simulink model "MMC_SIMULATION (1)"  (R2024a)
settings: Solver=ode1  StartTime=0.0  StopTime=2  FixedStep=1e-5  MaxStep=1e-5  RelTol=1e-5  EnableMultiTasking=on
InitFcn:
  | tau_iac=ts_G_iac/4;                                         %Current loop speed
  | wAC=1/tau_iac;                                              %Frequency
  | L1AC=wAC/s;                                                 %Open loop IMC (L) transfer function to obtain a first order after closing the loop
  | Kp_AC=wAC*(Lg_1+La_1/2);                                    %Proportional constant of the controller
  | Ki_AC=wAC*(Rg_1+Ra_1/2);                                    %Integral constant of the controller
  | C_IMC_AC=(Kp_AC*s+Ki_AC)/s;                                 %IMC designed PI controller transfer function
  | TAC=minreal((C_IMC_AC)*G_iac/(1+(C_IMC_AC)*G_iac));         %Closed loop transfer function
  | 
  | tau_Pac=ts_G_P/4;
  | D = TAC*U_ll1;
  | [C_pi,info] = pidtune(D,'PI',1/tau_Pac);
  | Ki_P = C_pi.Ki;
  | 
  | tau_Qac=ts_G_Q/4;
  | [C_piq,info] = pidtune(D,'PI',1/tau_Qac);
  | Ki_Q = C_piq.Ki;
  | 
  | 
  | tau_isum=ts_G_isum/4;                                        %Current loop speed
  | wsum=1/tau_isum;                                             %Frequency
  | L1AC=wsum/s;                                                 %Open loop IMC (L) transfer function to obtain a first order after closing the loop
  | Kp_sum=wsum*(2*La_1);                                        %Proportional constant of the controller
  | Ki_sum=wsum*(2*Ra_1);                                        %Integral constant of the controller
  | C_IMC_sum=(Kp_sum*s+Ki_sum)/s;                               %IMC designed PI controller transfer function
  | 
  | Kp_sum_PR = wc*(2*La_1);
  | Ki_sum_PR = wc*(2*Ra_1);
  | PR = (Kp_sum_PR*s^2 + 2*wc*(Kp_sum_PR+Ki_sum_PR)*s +Kp_sum_PR*w0^2)/(s^2+2*wc*s+w0^2);
  | 
  | 
  | %Energy reference for a converter arm (sum of all the submodule energies)
  | ArmEnergyRef=1/2*Carm*ArmVoltageRef^2;                      %Energy reference for a converter leg
  | LegEnergy=ArmEnergyRef*2;                                   %References for the controllers (DC side)
  | TotalEnergyRef=ArmEnergyRef*6;                              %Reference of the total energy of the converter
  | EnergyDiffabRef=0;                                          %Reference for the energy difference between legs a and b
  | EnergyDiffacRef=0;                                          %Reference for the energy difference between legs b and c
  | 
  | %References for the controllers (AC side)
  | EnergyDiffUpLowRefa=0;                                      %Reference for the energy difference upper and lower arms of phase a
  | EnergyDiffUpLowRefb=0;                                      %Reference for the energy difference upper and lower arms of phase b
  | EnergyDiffUpLowRefc=0;                                      %Reference for the energy difference upper and lower arms of phase c
  |                                                             %Controller design
  | Kpenergy=50;                                                %Proportional gain
  | Kienergy=20;                                                %Integral gain
  | 
  | Kpenergyt=50;                                               %Proportional gain
  | Kienergyt=20;                                               %Integral gain
  | 
  | Q=3;
  | wn=50*2*pi;                                                 %Frequency to eliminate 50 Hz
  | N_50 = tf([1 0 wn^2],[1 2*wn/Q wn^2]);                       %Notch filter 1 design
  | wn=100*2*pi;                                                %Frequency to eliminate 100 Hz
  | N_100 = tf([1 0 wn^2],[1 2*wn/Q wn^2]);                      %Notch filter 2 design
  | Notch=N_50*N_100;                                            %Combination of both notch filters
  | 
  | Ibasedc1= 1000e6/640e3;                 %Nominal current peak DC
  | IsaturationinnerDC1=1.1*Ibasedc1/3;  %Saturation of the DC inner current
  | IsaturationinnerAC1=0.45*Ibasedc1/3; %0.45  %Saturation of the inner current (why edu used 10% - FYI I changed it to 45%)
values from neighbouring files (symbols this model uses):
  ArmVoltageRef = 640e3    (= 640000)    [MMC_code.m]
  Cap = 9.5e-3    (= 0.0095)    [MMC_code.m]
  Carm = Cap/N    (= 2.375e-05)    [MMC_code.m]
  f_grid = 50    [MMC_code.m]
  G_iac = 1/((Lg_1+La_1/2)*s+(Rg_1+Ra_1/2))    [MMC_Parameters.m]    (also in MMC_code.m)
  La_1 = 0.15*Zbase_1/(2*pi*50)    (= 0.0488923985178)    [MMC_code.m]
  Lg_1 = 0.18*Zbase_1/(2*pi*50)    (= 0.0586708782214)    [MMC_code.m]
  N = 400    [MMC_code.m]
  Ra_1 = 0.01*Zbase_1    (= 1.024)    [MMC_code.m]
  Rg_1 = 0.005*Zbase_1    (= 0.512)    [MMC_code.m]
  s = tf('s')    [MMC_Parameters.m]    (also in MMC_code.m)
  S_1 = 1000e6    (= 1000000000)    [MMC_code.m]
  ts_G_iac = 10e-3    (= 0.01)    [MMC_Parameters.m]    (also in MMC_code.m)
  ts_G_isum = 1e-3    (= 0.001)    [MMC_Parameters.m]    (also in MMC_code.m)
  ts_G_P = 25e-3    (= 0.025)    [MMC_Parameters.m]    (also in MMC_code.m)
  ts_G_Q = 25e-3    (= 0.025)    [MMC_Parameters.m]    (also in MMC_code.m)
  U_ll1 = 320e3    (= 320000)    [MMC_code.m]
  Vdc = 640e3    (= 640000)    [MMC_code.m]
  Vpeak_d1 = U_pnpeak1    [MMC_code.m]
  w0 = 2*pi*f_grid    (= 314.159265359)    [MMC_code.m]
  wc = 2*pi*5    (= 31.4159265359)    [MMC_Parameters.m]    (also in MMC_code.m)
undefined symbols (not defined in the file or in its folder): Kp_Pac
libraries: spsCurrentMeasurementLib x15, spsSeriesRLCBranchLib x15, spsControlledVoltageSourceLib x9, slpidlib x7, spsControlledCurrentSourceLib x6, spsVoltageMeasurementLib x6, powerlib_extras x1, spsDCVoltageSourceLib x1, spspowerguiLib x1
(part 1 of 2)
settings Model: Creator=Ibrahim  LastModifiedBy=Dell
settings SolverCC: AlgebraicLoopSolver=TrustRegion
settings DataIOCC: LimitDataPoints=on  SaveFormat=Array  SignalLoggingSaveFormat=ModelDataLogs  ReturnWorkspaceOutputs=off
settings OptimizationCC: LifeSpan=inf
settings DebuggingCC: SolverPrmCheckMsg=warning  MultiTaskDSMMsg=warning  MultiTaskCondExecSysMsg=none  UnconnectedInputMsg=warning  UnconnectedOutputMsg=warning  UnconnectedLineMsg=warning  StrictBusMsg=ErrorOnBusTreatedAsVector  SFUnexpectedBacktrackingDiag=warning  SFNoUnconditionalDefaultTransitionDiag=warning  SFExecutionAtInitializationDiag=none  ArithmeticOperatorsInVariantConditions=warning
settings HardwareCC: ProdBitPerPointer=32  ProdBitPerSizeT=32  ProdBitPerPtrDiffT=32  ProdLargestAtomicFloat=None  ProdIntDivRoundTo=Undefined  ProdEndianess=Unspecified  ProdWordSize=32  ProdHWDeviceType=32-bit Generic
settings ModelReferenceCC: EnableRefExpFcnMdlSchedulingChecks=on  PropagateSignalLabelsOutOfModel=off
settings SFSimCC: SimUseLocalCustomCode=off  CustomCodeUndefinedFunction=UseInterfaceOnly
settings RTWCC: RTWUseLocalCustomCode=off  GPUComputeCapability=3.5  DLArmComputeVersion=19.05
settings CodeAppCC: StateflowObjectComments=on
settings GRTTargetCC: TargetLangStandard=C89/C90 (ANSI)
settings ConfigComp: CovMetricSettings=dw  CovSaveCumulativeToWorkspaceVar=on  CovSaveSingleToWorkspaceVar=on  CovExternalEMLEnable=off
settings SimscapeCC: SimscapeNormalizeSystem=off

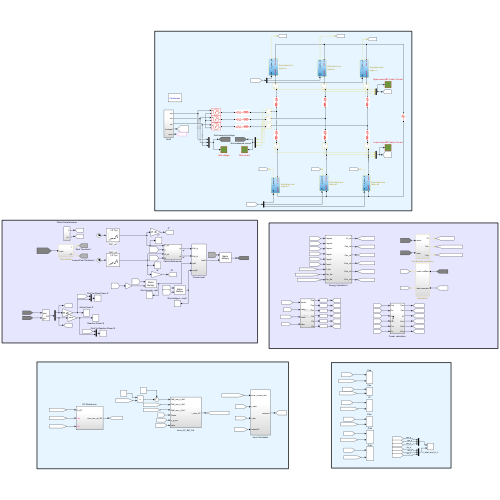
[thumbnail: Simulink's stored preview of the top-level diagram]
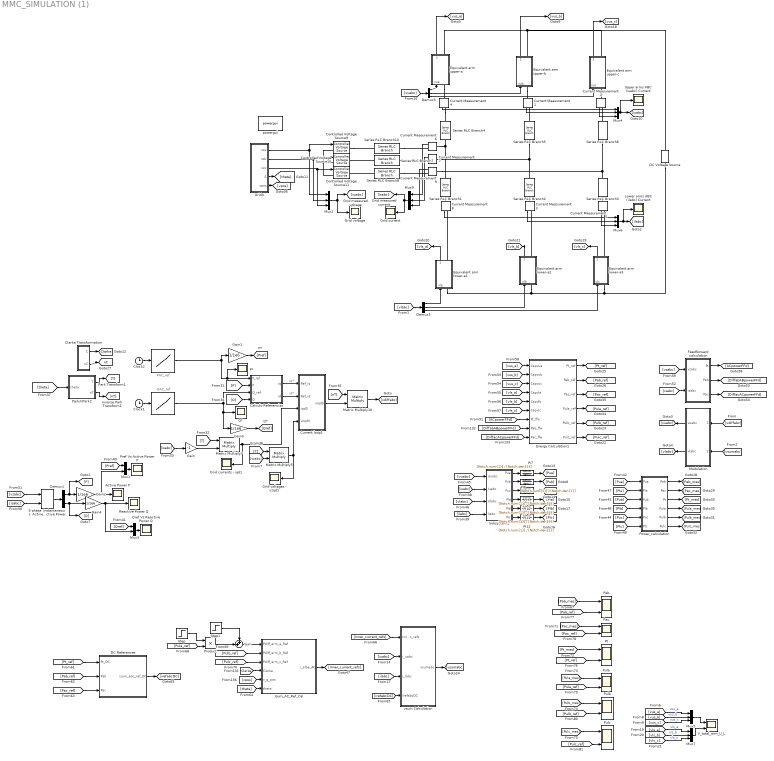
== system MMC_SIMULATION (1) ==
  note: PAC_ref
  note: QAC_ref
  " " : Lookup_n-D  NumberOfTableDimensions=1  BreakpointsForDimension1=[0,0.5,2]  Table=[0,100e6,0]  InterpMethod=Flat  RndMeth=Simplest
  "  " : Lookup_n-D  NumberOfTableDimensions=1  BreakpointsForDimension1=[0,1,2]  Table=[0,5e6,0]  InterpMethod=Flat  RndMeth=Simplest
  3-phase  Instantaneous  Active & Reactive Power : powerlib_extras/Measurements/3-phase  Instantaneous  Active & Reactive Power
  Active Power P : Scope
  Calculo Referencias : Subsystem
  "Clarke Transformation " : Subsystem
  Clock1 : Clock
  Clock2 : Clock
  Controlled Voltage Source10 : spsControlledVoltageSourceLib/Controlled Voltage Source  Initialize=off  Source_Type=AC  Amplitude=0  Phase=0  Frequency=0  Measurements=None
  Controlled Voltage Source11 : spsControlledVoltageSourceLib/Controlled Voltage Source  Initialize=off  Source_Type=AC  Amplitude=0  Phase=0  Frequency=0  Measurements=None
  Controlled Voltage Source9 : spsControlledVoltageSourceLib/Controlled Voltage Source  Initialize=off  Source_Type=AC  Amplitude=0  Phase=0  Frequency=0  Measurements=None
  Current Measurement{1..9} (9 alike) : spsCurrentMeasurementLib/Current Measurement  PhasorSimulation=off  OutputType=Complex  PSBequivalent=0
  Current loop1 : Subsystem
  DC References : Subsystem
  DC Voltage Source : spsDCVoltageSourceLib/DC Voltage Source  Amplitude=Vdc  Measurements=None
  Demux1 : Demux  Outputs=2
  Demux3 : Demux  Outputs=3
  Demux5 : Demux  Outputs=3
  Energy Calculation1 : Subsystem
  Equivalent arm lower-a1 : Subsystem
  Equivalent arm lower-a2 : Subsystem
  Equivalent arm lower-a3 : Subsystem
  Equivalent arm upper-a : Subsystem
  Equivalent arm upper-b : Subsystem
  Equivalent arm upper-c : Subsystem
  Feedforward calculation : Subsystem
  Gain : Gain  Gain=-1
  Gain{1..4} (4 alike) : Gain  Gain=1/1e6
  Grid current : Scope
  Grid currents - iqd1 : Scope
  Grid voltage : Scope
  Grid voltages - vzqd1 : Scope
  Grid3 : Subsystem
  Isum_AC_Ref_Cal : Subsystem
  Lower arms ABC (ilabc) Current : Scope
  Matrix Multiply10 : Product  Multiplication=Matrix(*)
  Matrix Multiply5 : Product  Multiplication=Matrix(*)
  Matrix Multiply7 : Product  Multiplication=Matrix(*)
  Modulation : Subsystem
  Mux1 : Mux  Inputs=2
  Mux{2,4..7,9} (6 alike) : Mux  Inputs=3
  Mux3 : Mux  Inputs=2
  P* : Scope
  PI{7..12} (6 alike) : TransferFcn  Numerator=[Notch.num{1}]  Denominator=[Notch.den{1}]
  Pab : Scope  NumInputPorts=2
  Pac : Scope  NumInputPorts=2
  Park/nPark2 : Subsystem
  Power_calculation : Subsystem
  Pref Vs Active Power P : Scope
  Product : Product
  Pt : Scope  NumInputPorts=2
  Pula : Scope  NumInputPorts=2
  Pulb : Scope  NumInputPorts=2
  Pulc : Scope  NumInputPorts=2
  Q* : Scope
  Qref Vs Reactive Power Q : Scope
  Reactive Power Q : Scope
  Series RLC Branch{1..6} (6 alike) : spsSeriesRLCBranchLib/Series RLC Branch  LConnTagsString=__new0  RConnTagsString=__new0  BranchType=RL  Resistance=Ra_1  Inductance=La_1  SetiL0=off  InitialCurrent=0  Capacitance=0  Setx0=off  InitialVoltage=0  Measurements=None
  Series RLC Branch10 : spsSeriesRLCBranchLib/Series RLC Branch  LConnTagsString=__new0  RConnTagsString=__new0  BranchType=RL  Resistance=Rg_1  Inductance=Lg_1  SetiL0=off  InitialCurrent=0  Capacitance=0  Setx0=off  InitialVoltage=0  Measurements=None
  Series RLC Branch7 : spsSeriesRLCBranchLib/Series RLC Branch  LConnTagsString=__new0  RConnTagsString=__new0  BranchType=RL  Resistance=Rg_1  Inductance=Lg_1  SetiL0=off  InitialCurrent=0  Capacitance=0  Setx0=off  InitialVoltage=0  Measurements=None
  Series RLC Branch8 : spsSeriesRLCBranchLib/Series RLC Branch  LConnTagsString=__new0  RConnTagsString=__new0  BranchType=RL  Resistance=Rg_1  Inductance=Lg_1  SetiL0=off  InitialCurrent=0  Capacitance=0  Setx0=off  InitialVoltage=0  Measurements=None
  Step : Step  Time=2.1  Before=1  After=0  SampleTime=0
  Step1 : Step  Time=2.1  After=10e6  SampleTime=0
  Subsystem1 : Subsystem
  Sum : Sum  Inputs=++|
  Upper arms ABC (iuabc) Current : Scope
  V_total_arm_U_L : Scope  NumInputPorts=2
  powergui : spspowerguiLib/powergui  Priority=1  SimulationMode=Continuous  SampleTime=50e-6  frequency=60  Iterations=50  frequencyindice=0  Pbase=100e6  ErrMax=1e-4  UnitsV=kV  UnitsW=MW  buscounter=0  FunctionMessages=off  echomessages=off  EnableUseOfTLC=off  CurrentSourceSwitches=on  DisableSnubberDevices=off  DisableRonSwitches=off  DisableVfSwitches=off  DisplayEquations=off  AutomaticDiscreteSolvers=off  SolverType=Tustin  Interpol=off  ExternalGateDelay=off  methode=off  Ts=0  x0status=blocks  SPID=off  SwTol=0  HookPort=off  NonlinearTolerance=1e-4  nMaxIteration=100  ContinueOnMaxIteration=off  RestoreLinks=warning  ResistiveCurrentMeasurement=off  Frange=[0:2:500]  Ylog=off  Xlog=on  ShowGrid=off  save=off  variable=ZData  structure=0  ZoomFFT=off  StartTime=0.0  cycles=1  DisplayStyle=1  fundamental=60  FreqAxis=off  MaxFrequency=1000  frequencyindicesteady=1  RmsSteady=1  display=off
  vsum Calculation : Subsystem
  tag scope: Clarke=global, nC=global
  wires:
  Mux4/1 -> Upper arms ABC (iuabc) Current/1, [iuabc]
  Grid3/4(thetareal) -> [theta]
  Grid3/1(vza) -> Controlled Voltage Source9/1, Mux2/1
  Grid3/2(vzb) -> Controlled Voltage Source10/1, Mux2/2
  Grid3/3(vzc) -> Controlled Voltage Source11/1, Mux2/3
  Mux2/1 -> [vzabc], Grid voltage/1
  Demux3/1 -> Equivalent arm lower-a1/1(vla)
  Demux3/2 -> Equivalent arm lower-a2/1(vlb)
  Demux3/3 -> Equivalent arm lower-a3/1(vlc)
  Mux6/1 -> Lower arms ABC (ilabc) Current/1, [ilabc]
  Current Measurement8/1 -> Mux6/1
  Current Measurement3/1 -> Mux6/2
  Current Measurement5/1 -> Mux6/3
  Modulation/1(vuabc) -> [vuabc]
  Modulation/2(vlabc) -> [vlabc]
  [vdiffabc] -> Modulation/1(vdiffabc)
  [vsumabc] -> Modulation/2(vsumabc)
  Current Measurement6/1 -> Mux9/1
  Current Measurement7/1 -> Mux9/2
  Current Measurement9/1 -> Mux9/3
  Mux9/1 -> [isabc], Grid current/1
  [vuabc] -> Demux5/1
  Demux5/1 -> Equivalent arm upper-a/1(vua)
  Demux5/2 -> Equivalent arm upper-b/1(vub)
  Demux5/3 -> Equivalent arm upper-c/1(vuc)
  [vlabc] -> Demux3/1
  Current Measurement4/1 -> Mux4/1
  Current Measurement1/1 -> Mux4/2
  Current Measurement2/1 -> Mux4/3
  [vls_c] -> Mux7/3  "vls_c"
  [vls_a] -> Mux7/1  "vls_a"
  [vls_b] -> Mux7/2  "vls_b"
  [vus_c] -> Mux5/3  "vus_c"
  [vus_a] -> Mux5/1  "vus_a"
  [vus_b] -> Mux5/2  "vus_b"
  Mux7/1 -> V_total_arm_U_L/2
  Mux5/1 -> V_total_arm_U_L/1
  Equivalent arm upper-c/1(v_sum_uc) -> [vus_c]
  Equivalent arm upper-b/1(v_sum_ub) -> [vus_b]
  Equivalent arm upper-a/1(v_sum_ua) -> [vus_a]
  Equivalent arm lower-a3/1(v_sum_lc) -> [vls_c]
  Equivalent arm lower-a2/1(v_sum_lb) -> [vls_b]
  Equivalent arm lower-a1/1(v_sum_la) -> [vls_a]
  Demux1/2 -> [Q], Gain4/1
  [vzabc] -> Matrix Multiply5/2
  [Pref] -> Mux1/1
  Calculo Referencias/1(iq) -> Current loop1/1(Ref_iq)  "iq*"
  Calculo Referencias/2(id) -> Current loop1/2(Ref_id)  "id*"
  [Qref] -> Mux3/1
  Matrix Multiply10/1 -> [vdiffabc]
  [T] -> Matrix Multiply7/1
  Gain/1 -> Matrix Multiply7/2
  Matrix Multiply7/1 -> Current loop1/3(iqd0), Grid currents - iqd1/1
  Demux1/1 -> [P], Gain2/1
  3-phase  Instantaneous  Active & Reactive Power/1 -> Demux1/1
  "  "/1 -> Calculo Referencias/3(Q_ref), Gain3/1, Q*/1
  Mux1/1 -> Pref Vs Active Power P/1
  Current loop1/1(vlqd0) -> Matrix Multiply10/2
  [T] -> Matrix Multiply5/1
  [isabc] -> Gain/1
  Gain2/1 -> Mux1/2, Active Power P/1
  [nT] -> Matrix Multiply10/1
  [theta] -> Park/nPark2/1(theta)
  Gain4/1 -> Mux3/2, Reactive Power Q/1
  Mux3/1 -> Qref Vs Reactive Power Q/1
  Park/nPark2/2("nT ") -> [nT]
  Gain1/1 -> [Pref]
  Park/nPark2/1(T) -> [T]
  Gain3/1 -> [Qref]
  Matrix Multiply5/1 -> Grid voltages - vzqd1/1, Current loop1/4(vzqd0)
  [P] -> Calculo Referencias/2(P)
  [Q] -> Calculo Referencias/4(Q)
  " "/1 -> P*/1, Calculo Referencias/1(P_ref), Gain1/1
  [isabc] -> 3-phase  Instantaneous  Active & Reactive Power/2
  [vzabc] -> 3-phase  Instantaneous  Active & Reactive Power/1
  [Pua] -> Power_calculation/1(Pua)
  [Pla] -> Power_calculation/2(Pla)
  [Pub] -> Power_calculation/3(Pub)
  [Plb] -> Power_calculation/4(Plb)
  [Puc] -> Power_calculation/5(Puc)
  [Plc] -> Power_calculation/6(Plc)
  [vuabc] -> Subsystem1/1(Uuabc)
  [iuabc] -> Subsystem1/2(Iuabc)
  [vlabc] -> Subsystem1/3(Ulabc)
  [ilabc] -> Subsystem1/4(Ilabc)
  Subsystem1/1(Pua) -> PI7/1
  Subsystem1/2(Pub) -> PI8/1
  Subsystem1/3(Puc) -> PI9/1
  Subsystem1/4(Pla) -> PI10/1
  Subsystem1/5(Plb) -> PI11/1
  Subsystem1/6(Plc) -> PI12/1
  Energy Calculation1/6(Pulc_ref) -> [Pulc_ref]
  [vls_b] -> Energy Calculation1/5(Capvlb)
  Energy Calculation1/1(Pt_ref) -> [Pt_ref]
  Energy Calculation1/3(Pac_ref) -> [Pac_ref]
  Energy Calculation1/2(Pab_ref) -> [Pab_ref]
  [vus_b] -> Energy Calculation1/2(Capvub)
  [vls_c] -> Energy Calculation1/6(Capvlc)
  Energy Calculation1/4(Pula_ref) -> [Pula_ref]
  Energy Calculation1/5(Pulb_ref) -> [Pulb_ref]
  [vus_a] -> Energy Calculation1/1(Capvua)
  [vls_a] -> Energy Calculation1/4(Capvla)
  [vus_c] -> Energy Calculation1/3(Capvuc)
  Feedforward calculation/2(Pab) -> [DiffabABpowerFFd]
  Feedforward calculation/3(Pac) -> [DiffacACpowerFFd]
  Feedforward calculation/1(Pt) -> [ACpowerFFd]
  [vzabc] -> Feedforward calculation/1(vzabc)
  [isabc] -> Feedforward calculation/2(isabc)
  [DiffacACpowerFFd] -> Energy Calculation1/9(Pac_ffw)
  [DiffabABpowerFFd] -> Energy Calculation1/8(Pab_ffw)
  [ACpowerFFd] -> Energy Calculation1/7(Pt_ffw)
  [Pt_ref] -> DC References/1(Pt_DC)
  [Pab_ref] -> DC References/2(Pab)
  [Pac_ref] -> DC References/3(Pac)
  [Pulc_ref] -> Isum_AC_Ref_Cal/3(Pdiff_arm_c_Ref)
  [Clarke] -> Isum_AC_Ref_Cal/4(Clarke)
  [Pulb_ref] -> Isum_AC_Ref_Cal/2(Pdiff_arm_b_Ref)
  [vpos] -> Isum_AC_Ref_Cal/5(v_g_pos)
  Isum_AC_Ref_Cal/1(i_albe_AC) -> [Inner_current_refs]
  DC References/1(isum_abc_ref_DC) -> [irefabcDC]
  [theta] -> Isum_AC_Ref_Cal/6(theta)
  vsum Calculation/1(vsumabc) -> [vsumabc]
  [ilabc] -> vsum Calculation/3(i_labc)
  [iuabc] -> vsum Calculation/2(i_uabc)
  [irefabcDC] -> vsum Calculation/4(irefabcDC)
  "Clarke Transformation "/2("nC ") -> [nC]
  "Clarke Transformation "/1(C) -> [Clarke]
  [Inner_current_refs] -> vsum Calculation/1(Inner_current_refs)
  [Pab_mes] -> Pab/1
  [Pab_ref] -> Pab/2
  [Pac_mes] -> Pac/1
  [Pac_ref] -> Pac/2
  [Pt_ref] -> Pt/2
  [Pt_mes] -> Pt/1
  [Pula_mes] -> Pula/1
  [Pula_ref] -> Pula/2
  [Pulb_mes] -> Pulb/1
  [Pulb_ref] -> Pulb/2
  [Pulc_mes] -> Pulc/1
  [Pulc_ref] -> Pulc/2
  Grid3/5(vpos) -> [vpos]
  Power_calculation/1(Pab) -> [Pab_mes]
  Power_calculation/2(Pac) -> [Pac_mes]
  Power_calculation/3(Pt) -> [Pt_mes]
  Power_calculation/4(Pula) -> [Pula_mes]
  Power_calculation/5(Pulb) -> [Pulb_mes]
  Power_calculation/6(Pulc) -> [Pulc_mes]
  PI7/1 -> [Pua]
  PI8/1 -> [Pub]
  PI9/1 -> [Puc]
  PI10/1 -> [Pla]
  PI11/1 -> [Plb]
  PI12/1 -> [Plc]
  Clock2/1 -> " "/1
  Clock1/1 -> "  "/1
  [Pula_ref] -> Product/2
  Product/1 -> Sum/2
  Step1/1 -> Sum/1
  Step/1 -> Product/1
  Sum/1 -> Isum_AC_Ref_Cal/1(Pdiff_arm_a_Ref)
  connections:
  Controlled Voltage Source9/LConn1 -- Controlled Voltage Source11/LConn1 -- Controlled Voltage Source10/LConn1
  Series RLC Branch4/RConn1 -- Series RLC Branch1/LConn1 -- Current Measurement6/LConn1
  DC Voltage Source/LConn1 -- Equivalent arm lower-a3/LConn1 -- Equivalent arm lower-a2/LConn1 -- Equivalent arm lower-a1/LConn1
  Series RLC Branch1/RConn1 -- Current Measurement8/LConn1
  Series RLC Branch2/RConn1 -- Current Measurement3/LConn1
  Series RLC Branch5/RConn1 -- Series RLC Branch2/LConn1 -- Current Measurement7/LConn1
  Series RLC Branch6/RConn1 -- Series RLC Branch3/LConn1 -- Current Measurement9/LConn1
  Series RLC Branch3/RConn1 -- Current Measurement5/LConn1
  Equivalent arm upper-a/LConn1 -- Current Measurement4/LConn1
  Current Measurement4/RConn1 -- Series RLC Branch4/LConn1
  Equivalent arm upper-b/LConn1 -- Current Measurement1/LConn1
  Series RLC Branch5/LConn1 -- Current Measurement1/RConn1
  Equivalent arm upper-c/LConn1 -- Current Measurement2/LConn1
  Series RLC Branch6/LConn1 -- Current Measurement2/RConn1
  Equivalent arm lower-a1/RConn1 -- Current Measurement8/RConn1
  Equivalent arm lower-a2/RConn1 -- Current Measurement3/RConn1
  Equivalent arm lower-a3/RConn1 -- Current Measurement5/RConn1
  Controlled Voltage Source9/RConn1 -- Series RLC Branch10/LConn1
  Series RLC Branch7/LConn1 -- Controlled Voltage Source10/RConn1
  Series RLC Branch8/LConn1 -- Controlled Voltage Source11/RConn1
  Series RLC Branch10/RConn1 -- Current Measurement6/RConn1
  Series RLC Branch7/RConn1 -- Current Measurement7/RConn1
  Series RLC Branch8/RConn1 -- Current Measurement9/RConn1
  DC Voltage Source/RConn1 -- Equivalent arm upper-c/RConn1 -- Equivalent arm upper-b/RConn1 -- Equivalent arm upper-a/RConn1

== system MMC_SIMULATION (1)/Calculo Referencias ==
  P_ref : Inport
  P : Inport  Port=2
  Q_ref : Inport  Port=3
  Q : Inport  Port=4
  Gain : Gain  Gain=-1
  Gain1 : Gain  Gain=-1
  PID Controller1 : slpidlib/PID Controller  Controller=I  Form=Parallel  TimeDomain=Continuous-time  UseExternalTs=off  SampleTime=1  IntegratorMethod=Forward Euler  FilterMethod=Forward Euler  ControllerParametersSource=internal  P=Kp_Pac  I=Ki_Q  UseKiTs=off  D=0  UseExternalDerivativeSource=off  N=100  UseFilter=on  TunerSelectOption=Transfer Function Based (PID Tuner App)  InitialConditionSource=internal  InitialConditionForIntegrator=0  InitialConditionForFilter=0  DifferentiatorICPrevScaledInput=0  ExternalReset=none  TrackingMode=off  Kt=1  LimitOutput=off  SatLimitsSource=internal  UpperSaturationLimit=inf  LowerSaturationLimit=-inf  LinearizeAsGain=on  AntiWindupMode=none  Kb=1  LimitIntegrator=off  UpperIntegratorSaturationLimit=inf  LowerIntegratorSaturationLimit=-inf  POutMin=[]  POutMax=[]  IOutMin=[]  IOutMax=[]  DOutMin=[]  DOutMax=[]  NOutMin=[]  NOutMax=[]  SumOutMin=[]  SumOutMax=[]  SaturationOutMin=[]  SaturationOutMax=[]  PParamMin=[]  PParamMax=[]  IParamMin=[]  IParamMax=[]  DParamMin=[]  DParamMax=[]  NParamMin=[]  NParamMax=[]  KbParamMin=[]  KbParamMax=[]  KtParamMin=[]  KtParamMax=[]  KbOutMin=[]  KbOutMax=[]  KtOutMin=[]  KtOutMax=[]  IntegratorOutMin=[]  IntegratorOutMax=[]  FilterOutMin=[]  FilterOutMax=[]  SumI1OutMin=[]  SumI1OutMax=[]  SumI2OutMin=[]  SumI2OutMax=[]  SumI3OutMin=[]  SumI3OutMax=[]  SumI4OutMin=[]  SumI4OutMax=[]  SumDOutMin=[]  SumDOutMax=[]  DifferentiatorOutMin=[]  DifferentiatorOutMax=[]  FilterDiffOutCoefMin=[]  FilterDiffOutCoefMax=[]  ReciprocalOutMin=[]  ReciprocalOutMax=[]  SumDenOutMin=[]  SumDenOutMax=[]  SumNumOutMin=[]  SumNumOutMax=[]  DivideOutMin=[]  DivideOutMax=[]  UdiffTsProdOutMin=[]  UdiffTsProdOutMax=[]  NTsProdOutMin=[]  NTsProdOutMax=[]  UintegralTsProdOutMin=[]  UintegralTsProdOutMax=[]  UngainTsProdOutMin=[]  UngainTsProdOutMax=[]  ClampingZeroOutDataTypeStr=Inherit: Inherit via back propagation  ClampingZeroOutMin=[]  ClampingZeroOutMax=[]  FilterDenConstantOutDataTypeStr=Inherit: Inherit via back propagation  FilterDenConstantOutMin=[]  FilterDenConstantOutMax=[]  PCopyOutDataTypeStr=Inherit: Inherit via back propagation  PCopyOutMin=[]  PCopyOutMax=[]  NCopyOutDataTypeStr=Inherit: Inherit via back propagation  NCopyOutMin=[]  NCopyOutMax=[]  IntegratorContinuousStateAttributes=''  IntegratorStateMustResolveToSignalObject=off  IntegratorRTWStateStorageClass=Auto  FilterContinuousStateAttributes=''  FilterStateMustResolveToSignalObject=off  FilterRTWStateStorageClass=Auto  ParallelPVariant=Disabled  IdealPVariant=Disabled  IVariant=InternalParameters  DVariant=Disabled  IntegratorVariant=Continuous  SatVariant=Disabled  AWVariant=Passthrough  PCopyVariant=Disabled  TRVariant=Disabled  FdbkBlocksVariant=Forward  IdealPFdbkVariant=Disabled  SatFdbkVariant=Disabled  DerivativeFilterVariant=Disabled  NVariant=Disabled  NCopyVariant=Disabled_SignalSpec  FilterICVariant=Disabled  IntegratorICVariant=InternalICs  ExternalResetVariant=Disabled  TRSumVariant=Passthrough  SumFdbkVariant=Disabled  SumVariant=Passthrough_I  TsampFilterVariant=InternalTs  TsampNgainVariant=Passthrough  TsampIntegralVariant=Disabled_SignalSpec  ExternalSaturationOutDataTypeStr=Inherit: Same as second input  DerivativeSourceVariant=Disabled
  PID Controller4 : slpidlib/PID Controller  Controller=I  Form=Parallel  TimeDomain=Continuous-time  UseExternalTs=off  SampleTime=1  IntegratorMethod=Forward Euler  FilterMethod=Forward Euler  ControllerParametersSource=internal  P=Kp_Pac  I=Ki_P  UseKiTs=off  D=0  UseExternalDerivativeSource=off  N=100  UseFilter=on  TunerSelectOption=Transfer Function Based (PID Tuner App)  InitialConditionSource=internal  InitialConditionForIntegrator=0  InitialConditionForFilter=0  DifferentiatorICPrevScaledInput=0  ExternalReset=none  TrackingMode=off  Kt=1  LimitOutput=off  SatLimitsSource=internal  UpperSaturationLimit=inf  LowerSaturationLimit=-inf  LinearizeAsGain=on  AntiWindupMode=none  Kb=1  LimitIntegrator=off  UpperIntegratorSaturationLimit=inf  LowerIntegratorSaturationLimit=-inf  POutMin=[]  POutMax=[]  IOutMin=[]  IOutMax=[]  DOutMin=[]  DOutMax=[]  NOutMin=[]  NOutMax=[]  SumOutMin=[]  SumOutMax=[]  SaturationOutMin=[]  SaturationOutMax=[]  PParamMin=[]  PParamMax=[]  IParamMin=[]  IParamMax=[]  DParamMin=[]  DParamMax=[]  NParamMin=[]  NParamMax=[]  KbParamMin=[]  KbParamMax=[]  KtParamMin=[]  KtParamMax=[]  KbOutMin=[]  KbOutMax=[]  KtOutMin=[]  KtOutMax=[]  IntegratorOutMin=[]  IntegratorOutMax=[]  FilterOutMin=[]  FilterOutMax=[]  SumI1OutMin=[]  SumI1OutMax=[]  SumI2OutMin=[]  SumI2OutMax=[]  SumI3OutMin=[]  SumI3OutMax=[]  SumI4OutMin=[]  SumI4OutMax=[]  SumDOutMin=[]  SumDOutMax=[]  DifferentiatorOutMin=[]  DifferentiatorOutMax=[]  FilterDiffOutCoefMin=[]  FilterDiffOutCoefMax=[]  ReciprocalOutMin=[]  ReciprocalOutMax=[]  SumDenOutMin=[]  SumDenOutMax=[]  SumNumOutMin=[]  SumNumOutMax=[]  DivideOutMin=[]  DivideOutMax=[]  UdiffTsProdOutMin=[]  UdiffTsProdOutMax=[]  NTsProdOutMin=[]  NTsProdOutMax=[]  UintegralTsProdOutMin=[]  UintegralTsProdOutMax=[]  UngainTsProdOutMin=[]  UngainTsProdOutMax=[]  ClampingZeroOutDataTypeStr=Inherit: Inherit via back propagation  ClampingZeroOutMin=[]  ClampingZeroOutMax=[]  FilterDenConstantOutDataTypeStr=Inherit: Inherit via back propagation  FilterDenConstantOutMin=[]  FilterDenConstantOutMax=[]  PCopyOutDataTypeStr=Inherit: Inherit via back propagation  PCopyOutMin=[]  PCopyOutMax=[]  NCopyOutDataTypeStr=Inherit: Inherit via back propagation  NCopyOutMin=[]  NCopyOutMax=[]  IntegratorContinuousStateAttributes=''  IntegratorStateMustResolveToSignalObject=off  IntegratorRTWStateStorageClass=Auto  FilterContinuousStateAttributes=''  FilterStateMustResolveToSignalObject=off  FilterRTWStateStorageClass=Auto  ParallelPVariant=Disabled  IdealPVariant=Disabled  IVariant=InternalParameters  DVariant=Disabled  IntegratorVariant=Continuous  SatVariant=Disabled  AWVariant=Passthrough  PCopyVariant=Disabled  TRVariant=Disabled  FdbkBlocksVariant=Forward  IdealPFdbkVariant=Disabled  SatFdbkVariant=Disabled  DerivativeFilterVariant=Disabled  NVariant=Disabled  NCopyVariant=Disabled_SignalSpec  FilterICVariant=Disabled  IntegratorICVariant=InternalICs  ExternalResetVariant=Disabled  TRSumVariant=Passthrough  SumFdbkVariant=Disabled  SumVariant=Passthrough_I  TsampFilterVariant=InternalTs  TsampNgainVariant=Passthrough  TsampIntegralVariant=Disabled_SignalSpec  ExternalSaturationOutDataTypeStr=Inherit: Same as second input  DerivativeSourceVariant=Disabled
  Sum1 : Sum  Inputs=|+-
  Sum5 : Sum  Inputs=|+-
  iq : Outport
  id : Outport  Port=2
  wires:
  P_ref/1 -> Sum5/1
  P/1 -> Sum5/2
  Sum5/1 -> PID Controller4/1
  PID Controller4/1 -> Gain/1
  Sum1/1 -> PID Controller1/1
  Q_ref/1 -> Sum1/1
  Q/1 -> Sum1/2
  PID Controller1/1 -> Gain1/1
  Gain/1 -> iq/1
  Gain1/1 -> id/1

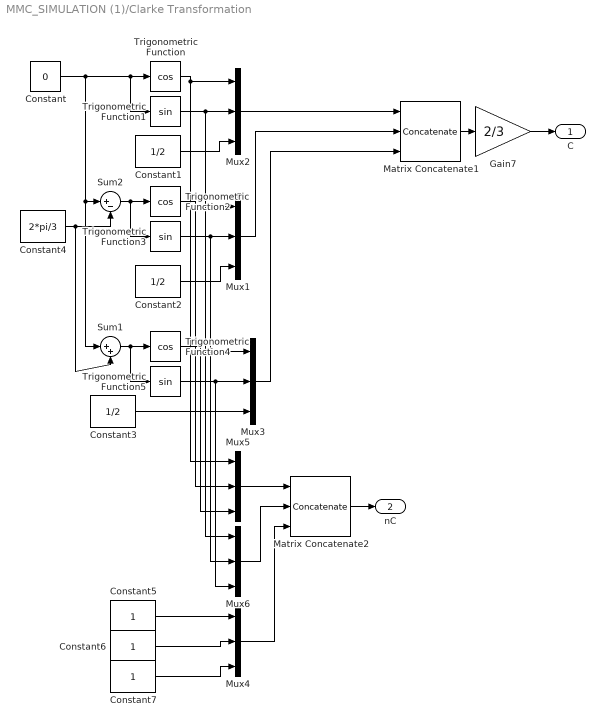
== system MMC_SIMULATION (1)/Clarke Transformation  ==
  Constant : Constant  Value=0
  Constant1 : Constant  Value=1/2  SampleTime=0
  Constant2 : Constant  Value=1/2  SampleTime=0
  Constant3 : Constant  Value=1/2  SampleTime=0
  Constant4 : Constant  Value=2*pi/3  SampleTime=0
  Constant5 : Constant  SampleTime=0
  Constant6 : Constant  SampleTime=0
  Constant7 : Constant  SampleTime=0
  Gain7 : Gain  Gain=2/3
  Matrix Concatenate1 : Concatenate  NumInputs=3  Mode=Multidimensional array  ConcatenateDimension=2
  Matrix Concatenate2 : Concatenate  NumInputs=3  Mode=Multidimensional array  ConcatenateDimension=2
  Mux{1..6} (6 alike) : Mux  Inputs=3
  Sum1 : Sum  Inputs=|++
  Sum2 : Sum  Inputs=|+-
  Trigonometric Function : Trigonometry  Operator=cos
  Trigonometric Function1 : Trigonometry
  Trigonometric Function2 : Trigonometry  Operator=cos
  Trigonometric Function3 : Trigonometry
  Trigonometric Function4 : Trigonometry  Operator=cos
  Trigonometric Function5 : Trigonometry
  C : Outport  VectorParamsAs1DForOutWhenUnconnected=off
  "nC " : Outport  Port=2  VectorParamsAs1DForOutWhenUnconnected=off
  wires:
  Matrix Concatenate2/1 -> "nC "/1
  Gain7/1 -> C/1
  Constant/1 -> Trigonometric Function1/1, Trigonometric Function/1, Sum2/1, Sum1/1
  Mux6/1 -> Matrix Concatenate2/2
  Mux5/1 -> Matrix Concatenate2/1
  Matrix Concatenate1/1 -> Gain7/1
  Mux3/1 -> Matrix Concatenate1/3
  Mux1/1 -> Matrix Concatenate1/2
  Mux2/1 -> Matrix Concatenate1/1
  Trigonometric Function5/1 -> Mux3/2, Mux6/3
  Trigonometric Function4/1 -> Mux5/3, Mux3/1
  Trigonometric Function3/1 -> Mux1/2, Mux6/2
  Trigonometric Function2/1 -> Mux1/1, Mux5/2
  Trigonometric Function1/1 -> Mux6/1, Mux2/2
  Trigonometric Function/1 -> Mux5/1, Mux2/1
  Constant4/1 -> Sum1/2, Sum2/2
  Sum1/1 -> Trigonometric Function5/1, Trigonometric Function4/1
  Sum2/1 -> Trigonometric Function3/1, Trigonometric Function2/1
  Constant1/1 -> Mux2/3
  Constant2/1 -> Mux1/3
  Constant3/1 -> Mux3/3
  Constant5/1 -> Mux4/1
  Constant6/1 -> Mux4/2
  Constant7/1 -> Mux4/3
  Mux4/1 -> Matrix Concatenate2/3

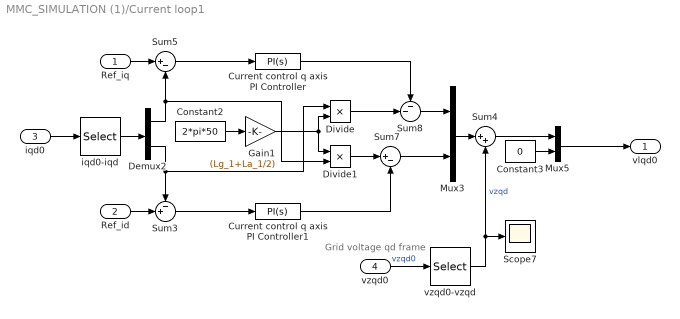
== system MMC_SIMULATION (1)/Current loop1 ==
  note: Grid voltage qd frame
  Ref_iq : Inport
  Ref_id : Inport  Port=2
  iqd0 : Inport  Port=3
  vzqd0 : Inport  Port=4
  Constant2 : Constant  Value=2*pi*50  SampleTime=-1
  Constant3 : Constant  Value=0
  Current control q axis PI Controller : slpidlib/PID Controller  Controller=PI  Form=Parallel  TimeDomain=Continuous-time  UseExternalTs=off  SampleTime=1  IntegratorMethod=Forward Euler  FilterMethod=Forward Euler  ControllerParametersSource=internal  P=Kp_AC  I=Ki_AC  UseKiTs=off  D=0  UseExternalDerivativeSource=off  N=100  UseFilter=on  TunerSelectOption=Transfer Function Based (PID Tuner App)  InitialConditionSource=internal  InitialConditionForIntegrator=0  InitialConditionForFilter=0  DifferentiatorICPrevScaledInput=0  ExternalReset=none  TrackingMode=off  Kt=1  LimitOutput=off  SatLimitsSource=internal  UpperSaturationLimit=inf  LowerSaturationLimit=-inf  LinearizeAsGain=on  AntiWindupMode=none  Kb=1  LimitIntegrator=off  UpperIntegratorSaturationLimit=inf  LowerIntegratorSaturationLimit=-inf  POutMin=[]  POutMax=[]  IOutMin=[]  IOutMax=[]  DOutMin=[]  DOutMax=[]  NOutMin=[]  NOutMax=[]  SumOutMin=[]  SumOutMax=[]  SaturationOutMin=[]  SaturationOutMax=[]  PParamMin=[]  PParamMax=[]  IParamMin=[]  IParamMax=[]  DParamMin=[]  DParamMax=[]  NParamMin=[]  NParamMax=[]  KbParamMin=[]  KbParamMax=[]  KtParamMin=[]  KtParamMax=[]  KbOutMin=[]  KbOutMax=[]  KtOutMin=[]  KtOutMax=[]  IntegratorOutMin=[]  IntegratorOutMax=[]  FilterOutMin=[]  FilterOutMax=[]  SumI1OutMin=[]  SumI1OutMax=[]  SumI2OutMin=[]  SumI2OutMax=[]  SumI3OutMin=[]  SumI3OutMax=[]  SumI4OutMin=[]  SumI4OutMax=[]  SumDOutMin=[]  SumDOutMax=[]  DifferentiatorOutMin=[]  DifferentiatorOutMax=[]  FilterDiffOutCoefMin=[]  FilterDiffOutCoefMax=[]  ReciprocalOutMin=[]  ReciprocalOutMax=[]  SumDenOutMin=[]  SumDenOutMax=[]  SumNumOutMin=[]  SumNumOutMax=[]  DivideOutMin=[]  DivideOutMax=[]  UdiffTsProdOutMin=[]  UdiffTsProdOutMax=[]  NTsProdOutMin=[]  NTsProdOutMax=[]  UintegralTsProdOutMin=[]  UintegralTsProdOutMax=[]  UngainTsProdOutMin=[]  UngainTsProdOutMax=[]  ClampingZeroOutDataTypeStr=Inherit: Inherit via back propagation  ClampingZeroOutMin=[]  ClampingZeroOutMax=[]  FilterDenConstantOutDataTypeStr=Inherit: Inherit via back propagation  FilterDenConstantOutMin=[]  FilterDenConstantOutMax=[]  PCopyOutDataTypeStr=Inherit: Inherit via back propagation  PCopyOutMin=[]  PCopyOutMax=[]  NCopyOutDataTypeStr=Inherit: Inherit via back propagation  NCopyOutMin=[]  NCopyOutMax=[]  IntegratorContinuousStateAttributes=''  IntegratorStateMustResolveToSignalObject=off  IntegratorRTWStateStorageClass=Auto  FilterContinuousStateAttributes=''  FilterStateMustResolveToSignalObject=off  FilterRTWStateStorageClass=Auto  ParallelPVariant=InternalParameters  IdealPVariant=Disabled  IVariant=InternalParameters  DVariant=Disabled  IntegratorVariant=Continuous  SatVariant=Disabled  AWVariant=Passthrough  PCopyVariant=Disabled  TRVariant=Disabled  FdbkBlocksVariant=Forward  IdealPFdbkVariant=Disabled  SatFdbkVariant=Disabled  DerivativeFilterVariant=Disabled  NVariant=Disabled  NCopyVariant=Disabled_SignalSpec  FilterICVariant=Disabled  IntegratorICVariant=InternalICs  ExternalResetVariant=Disabled  TRSumVariant=Passthrough  SumFdbkVariant=Disabled  SumVariant=Sum_PI  TsampFilterVariant=InternalTs  TsampNgainVariant=Passthrough  TsampIntegralVariant=Disabled_SignalSpec  ExternalSaturationOutDataTypeStr=Inherit: Same as second input  DerivativeSourceVariant=Disabled
  Current control q axis PI Controller1 : slpidlib/PID Controller  Controller=PI  Form=Parallel  TimeDomain=Continuous-time  UseExternalTs=off  SampleTime=1  IntegratorMethod=Forward Euler  FilterMethod=Forward Euler  ControllerParametersSource=internal  P=Kp_AC  I=Ki_AC  UseKiTs=off  D=0  UseExternalDerivativeSource=off  N=100  UseFilter=on  TunerSelectOption=Transfer Function Based (PID Tuner App)  InitialConditionSource=internal  InitialConditionForIntegrator=0  InitialConditionForFilter=0  DifferentiatorICPrevScaledInput=0  ExternalReset=none  TrackingMode=off  Kt=1  LimitOutput=off  SatLimitsSource=internal  UpperSaturationLimit=inf  LowerSaturationLimit=-inf  LinearizeAsGain=on  AntiWindupMode=none  Kb=1  LimitIntegrator=off  UpperIntegratorSaturationLimit=inf  LowerIntegratorSaturationLimit=-inf  POutMin=[]  POutMax=[]  IOutMin=[]  IOutMax=[]  DOutMin=[]  DOutMax=[]  NOutMin=[]  NOutMax=[]  SumOutMin=[]  SumOutMax=[]  SaturationOutMin=[]  SaturationOutMax=[]  PParamMin=[]  PParamMax=[]  IParamMin=[]  IParamMax=[]  DParamMin=[]  DParamMax=[]  NParamMin=[]  NParamMax=[]  KbParamMin=[]  KbParamMax=[]  KtParamMin=[]  KtParamMax=[]  KbOutMin=[]  KbOutMax=[]  KtOutMin=[]  KtOutMax=[]  IntegratorOutMin=[]  IntegratorOutMax=[]  FilterOutMin=[]  FilterOutMax=[]  SumI1OutMin=[]  SumI1OutMax=[]  SumI2OutMin=[]  SumI2OutMax=[]  SumI3OutMin=[]  SumI3OutMax=[]  SumI4OutMin=[]  SumI4OutMax=[]  SumDOutMin=[]  SumDOutMax=[]  DifferentiatorOutMin=[]  DifferentiatorOutMax=[]  FilterDiffOutCoefMin=[]  FilterDiffOutCoefMax=[]  ReciprocalOutMin=[]  ReciprocalOutMax=[]  SumDenOutMin=[]  SumDenOutMax=[]  SumNumOutMin=[]  SumNumOutMax=[]  DivideOutMin=[]  DivideOutMax=[]  UdiffTsProdOutMin=[]  UdiffTsProdOutMax=[]  NTsProdOutMin=[]  NTsProdOutMax=[]  UintegralTsProdOutMin=[]  UintegralTsProdOutMax=[]  UngainTsProdOutMin=[]  UngainTsProdOutMax=[]  ClampingZeroOutDataTypeStr=Inherit: Inherit via back propagation  ClampingZeroOutMin=[]  ClampingZeroOutMax=[]  FilterDenConstantOutDataTypeStr=Inherit: Inherit via back propagation  FilterDenConstantOutMin=[]  FilterDenConstantOutMax=[]  PCopyOutDataTypeStr=Inherit: Inherit via back propagation  PCopyOutMin=[]  PCopyOutMax=[]  NCopyOutDataTypeStr=Inherit: Inherit via back propagation  NCopyOutMin=[]  NCopyOutMax=[]  IntegratorContinuousStateAttributes=''  IntegratorStateMustResolveToSignalObject=off  IntegratorRTWStateStorageClass=Auto  FilterContinuousStateAttributes=''  FilterStateMustResolveToSignalObject=off  FilterRTWStateStorageClass=Auto  ParallelPVariant=InternalParameters  IdealPVariant=Disabled  IVariant=InternalParameters  DVariant=Disabled  IntegratorVariant=Continuous  SatVariant=Disabled  AWVariant=Passthrough  PCopyVariant=Disabled  TRVariant=Disabled  FdbkBlocksVariant=Forward  IdealPFdbkVariant=Disabled  SatFdbkVariant=Disabled  DerivativeFilterVariant=Disabled  NVariant=Disabled  NCopyVariant=Disabled_SignalSpec  FilterICVariant=Disabled  IntegratorICVariant=InternalICs  ExternalResetVariant=Disabled  TRSumVariant=Passthrough  SumFdbkVariant=Disabled  SumVariant=Sum_PI  TsampFilterVariant=InternalTs  TsampNgainVariant=Passthrough  TsampIntegralVariant=Disabled_SignalSpec  ExternalSaturationOutDataTypeStr=Inherit: Same as second input  DerivativeSourceVariant=Disabled
  Demux2 : Demux  Outputs=2
  Divide : Product  Inputs=**
  Divide1 : Product  Inputs=**
  Gain1 : Gain  Gain=(Lg_1+La_1/2)
  Mux3 : Mux  Inputs=2
  Mux5 : Mux  Inputs=2
  Scope7 : Scope
  Sum3 : Sum  Inputs=-+|
  Sum4 : Sum  Inputs=|++
  Sum5 : Sum  Inputs=|+-
  Sum7 : Sum  Inputs=|+-
  Sum8 : Sum  Inputs=--|
  iqd0-iqd : Selector  InputPortWidth=3  IndexOptions=Index vector (dialog)  Indices=[1 2]  OutputSizes=1
  vzqd0-vzqd : Selector  InputPortWidth=3  IndexOptions=Index vector (dialog)  Indices=[1 2]  OutputSizes=1
  vlqd0 : Outport
  wires:
  Ref_iq/1 -> Sum5/1
  Ref_id/1 -> Sum3/2
  Current control q axis PI Controller/1 -> Sum8/1
  Mux3/1 -> Sum4/1
  vzqd0-vzqd/1 -> Scope7/1, Sum4/2  "vzqd"
  Sum5/1 -> Current control q axis PI Controller/1
  Gain1/1 -> Divide1/1, Divide/2
  Constant2/1 -> Gain1/1
  Demux2/1 -> Divide1/2, Sum5/2
  Divide/1 -> Sum8/2
  vzqd0/1 -> vzqd0-vzqd/1  "vzqd0"
  Sum4/1 -> Mux5/1
  Sum7/1 -> Mux3/2
  Sum3/1 -> Current control q axis PI Controller1/1
  Divide1/1 -> Sum7/1
  Sum8/1 -> Mux3/1
  Current control q axis PI Controller1/1 -> Sum7/2
  Constant3/1 -> Mux5/2
  Demux2/2 -> Sum3/1, Divide/1
  iqd0/1 -> iqd0-iqd/1
  iqd0-iqd/1 -> Demux2/1
  Mux5/1 -> vlqd0/1

== system MMC_SIMULATION (1)/DC References ==
  Pt_DC : Inport
  Pab : Inport  Port=2
  Pac : Inport  Port=3
  Constant : Constant  Value=[1,1,1;1,-2,1;1,1,-2]
  Gain1 : Gain  Gain=1/(3*Vdc)
  Matrix Multiply2 : Product  Multiplication=Matrix(*)
  Mux10 : Mux  Inputs=3
  Sat3 : Subsystem
  isum_abc_ref_DC : Outport
  wires:
  Matrix Multiply2/1 -> Gain1/1
  Constant/1 -> Matrix Multiply2/1
  Mux10/1 -> Matrix Multiply2/2
  Gain1/1 -> Sat3/1(In1)  "isum_abc_ref_DC"
  Pt_DC/1 -> Mux10/1
  Pac/1 -> Mux10/3
  Pab/1 -> Mux10/2
  Sat3/1(Out1) -> isum_abc_ref_DC/1

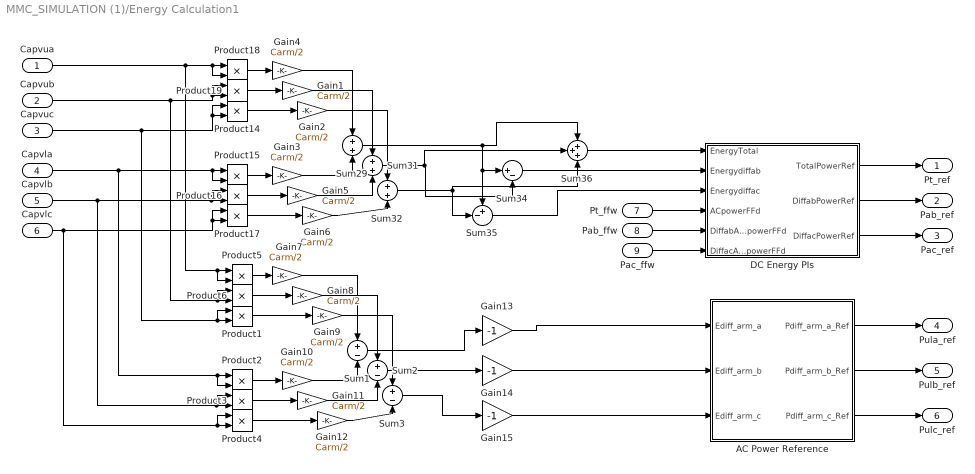
== system MMC_SIMULATION (1)/Energy Calculation1 ==
  Capvua : Inport
  Capvub : Inport  Port=2
  Capvuc : Inport  Port=3
  Capvla : Inport  Port=4
  Capvlb : Inport  Port=5
  Capvlc : Inport  Port=6
  Pt_ffw : Inport  Port=7
  Pab_ffw : Inport  Port=8
  Pac_ffw : Inport  Port=9
  AC Power Reference : Subsystem
  DC Energy PIs : Subsystem
  Gain{1..12} (12 alike) : Gain  Gain=Carm/2
  Gain13 : Gain  Gain=-1
  Gain14 : Gain  Gain=-1
  Gain15 : Gain  Gain=-1
  Product{1..6,14..19} (12 alike) : Product
  Sum1 : Sum  Inputs=+-
  Sum2 : Sum  Inputs=+-
  Sum29 : Sum
  Sum3 : Sum  Inputs=+-
  Sum31 : Sum
  Sum32 : Sum
  Sum34 : Sum  Inputs=|+-
  Sum35 : Sum  Inputs=+-|
  Sum36 : Sum  Inputs=+++
  Pt_ref : Outport
  Pab_ref : Outport  Port=2
  Pac_ref : Outport  Port=3
  Pula_ref : Outport  Port=4
  Pulb_ref : Outport  Port=5
  Pulc_ref : Outport  Port=6
  wires:
  Product6/1 -> Gain8/1
  Product4/1 -> Gain12/1
  Product2/1 -> Gain10/1
  Product1/1 -> Gain9/1
  Product3/1 -> Gain11/1
  Product5/1 -> Gain7/1
  Sum32/1 -> Sum36/3, Sum35/2
  Sum36/1 -> DC Energy PIs/1(EnergyTotal)
  Sum35/1 -> DC Energy PIs/3(Energydiffac)
  Sum34/1 -> DC Energy PIs/2(Energydiffab)
  Product19/1 -> Gain1/1
  Sum31/1 -> Sum36/2, Sum34/2
  Product17/1 -> Gain6/1
  Sum29/1 -> Sum35/1, Sum34/1, Sum36/1
  Product15/1 -> Gain3/1
  Product14/1 -> Gain2/1
  Product16/1 -> Gain5/1
  Product18/1 -> Gain4/1
  Capvlb/1 -> Product16/2, Product16/1, Product3/2, Product3/1
  Capvub/1 -> Product19/2, Product19/1, Product6/2, Product6/1
  Capvuc/1 -> Product14/2, Product14/1, Product1/2, Product1/1
  Capvua/1 -> Product18/1, Product18/2, Product5/1, Product5/2
  Capvla/1 -> Product15/1, Product15/2, Product2/1, Product2/2
  Capvlc/1 -> Product17/2, Product17/1, Product4/2, Product4/1
  Gain4/1 -> Sum29/1
  Gain1/1 -> Sum31/1
  Gain2/1 -> Sum32/1
  Gain9/1 -> Sum3/1
  Gain8/1 -> Sum2/1
  Gain7/1 -> Sum1/1
  Gain3/1 -> Sum29/2
  Gain5/1 -> Sum31/2
  Gain6/1 -> Sum32/2
  Gain10/1 -> Sum1/2
  Gain12/1 -> Sum3/2
  Gain11/1 -> Sum2/2
  Sum1/1 -> Gain13/1
  Sum2/1 -> Gain14/1
  Sum3/1 -> Gain15/1
  Pt_ffw/1 -> DC Energy PIs/4(ACpowerFFd)
  Pab_ffw/1 -> DC Energy PIs/5(DiffabABpowerFFd)
  Pac_ffw/1 -> DC Energy PIs/6(DiffacACpowerFFd)
  DC Energy PIs/1(TotalPowerRef) -> Pt_ref/1
  DC Energy PIs/3(DiffacPowerRef) -> Pac_ref/1
  DC Energy PIs/2(DiffabPowerRef) -> Pab_ref/1
  AC Power Reference/1(Pdiff_arm_a_Ref) -> Pula_ref/1
  AC Power Reference/2(Pdiff_arm_b_Ref) -> Pulb_ref/1
  AC Power Reference/3(Pdiff_arm_c_Ref) -> Pulc_ref/1
  Gain13/1 -> AC Power Reference/1(Ediff_arm_a)
  Gain15/1 -> AC Power Reference/3(Ediff_arm_c)
  Gain14/1 -> AC Power Reference/2(Ediff_arm_b)

== system MMC_SIMULATION (1)/Equivalent arm lower-a1 ==
  note: Power_la
  vla : Inport
  Controlled Current Source : spsControlledCurrentSourceLib/Controlled Current Source  Initialize=on  Source_Type=AC  Amplitude=0  Phase=0  Frequency=0  Measurements=None
  Controlled Voltage Source7 : spsControlledVoltageSourceLib/Controlled Voltage Source  Initialize=on  Source_Type=AC  Amplitude=Vdc/2  Phase=0  Frequency=0  Measurements=None
  Current Measurement4 : spsCurrentMeasurementLib/Current Measurement  PhasorSimulation=off  OutputType=Complex  PSBequivalent=0
  Divide1 : Product  Inputs=**
  Divide2 : Product  Inputs=*/
  Filtered Lower arm A instananeous power1 : Scope
  Gain : Gain  Gain=1e6
  Lower arm A instananeous power : Scope
  Series RLC Branch2 : spsSeriesRLCBranchLib/Series RLC Branch  LConnTagsString=__new0  RConnTagsString=__new0  BranchType=C  Resistance=Ra_1  Inductance=La_1  SetiL0=on  InitialCurrent=0  Capacitance=Cap/N  Setx0=on  InitialVoltage=640e3  Measurements=None
  Transfer Fcn : TransferFcn  Denominator=[1 1]
  Voltage Measurement : spsVoltageMeasurementLib/Voltage Measurement  PhasorSimulation=off  OutputType=Complex  PSBequivalent=0
  Conn1 : PMIOPort  Side=Right
  Conn2 : PMIOPort  Port=2  Side=Left
  v_sum_la : Outport
  wires:
  Gain/1 -> Filtered Lower arm A instananeous power1/1
  Transfer Fcn/1 -> Gain/1
  Current Measurement4/1 -> Divide1/2  "ila"
  Divide1/1 -> Divide2/1, Transfer Fcn/1, Lower arm A instananeous power/1
  Divide2/1 -> Controlled Current Source/1
  Voltage Measurement/1 -> Divide2/2, v_sum_la/1
  vla/1 -> Controlled Voltage Source7/1, Divide1/1  "vla"
  connections:
  Conn2/RConn1 -- Current Measurement4/RConn1
  Current Measurement4/LConn1 -- Controlled Voltage Source7/LConn1
  Voltage Measurement/LConn2 -- Series RLC Branch2/RConn1 -- Controlled Current Source/LConn1
  Controlled Current Source/RConn1 -- Series RLC Branch2/LConn1 -- Voltage Measurement/LConn1
  Controlled Voltage Source7/RConn1 -- Conn1/RConn1

== system MMC_SIMULATION (1)/Equivalent arm lower-a2 ==
  note: Power_lb
  vlb : Inport
  Controlled Current Source : spsControlledCurrentSourceLib/Controlled Current Source  Initialize=on  Source_Type=AC  Amplitude=0  Phase=0  Frequency=0  Measurements=None
  Controlled Voltage Source7 : spsControlledVoltageSourceLib/Controlled Voltage Source  Initialize=on  Source_Type=AC  Amplitude=Vdc/2  Phase=0  Frequency=0  Measurements=None
  Current Measurement4 : spsCurrentMeasurementLib/Current Measurement  PhasorSimulation=off  OutputType=Complex  PSBequivalent=0
  Divide1 : Product  Inputs=**
  Divide2 : Product  Inputs=*/
  Filtered Lower arm B instananeous power1 : Scope
  Gain : Gain  Gain=1e6
  Lower arm B instananeous power : Scope
  Series RLC Branch2 : spsSeriesRLCBranchLib/Series RLC Branch  LConnTagsString=__new0  RConnTagsString=__new0  BranchType=C  Resistance=Ra_1  Inductance=La_1  SetiL0=on  InitialCurrent=0  Capacitance=Cap/N  Setx0=on  InitialVoltage=640e3  Measurements=None
  Transfer Fcn : TransferFcn  Denominator=[1 1]
  Voltage Measurement : spsVoltageMeasurementLib/Voltage Measurement  PhasorSimulation=off  OutputType=Complex  PSBequivalent=0
  Conn1 : PMIOPort  Side=Right
  Conn2 : PMIOPort  Port=2  Side=Left
  v_sum_lb : Outport
  wires:
  vlb/1 -> Divide1/1, Controlled Voltage Source7/1  "vlb"
  Voltage Measurement/1 -> v_sum_lb/1, Divide2/2
  Divide2/1 -> Controlled Current Source/1
  Divide1/1 -> Lower arm B instananeous power/1, Transfer Fcn/1, Divide2/1
  Current Measurement4/1 -> Divide1/2  "ilb"
  Transfer Fcn/1 -> Gain/1
  Gain/1 -> Filtered Lower arm B instananeous power1/1
  connections:
  Controlled Voltage Source7/RConn1 -- Conn1/RConn1
  Voltage Measurement/LConn1 -- Series RLC Branch2/LConn1 -- Controlled Current Source/RConn1
  Controlled Current Source/LConn1 -- Series RLC Branch2/RConn1 -- Voltage Measurement/LConn2
  Current Measurement4/LConn1 -- Controlled Voltage Source7/LConn1
  Conn2/RConn1 -- Current Measurement4/RConn1

== system MMC_SIMULATION (1)/Equivalent arm lower-a3 ==
  note: Power_lc
  vlc : Inport
  Controlled Current Source : spsControlledCurrentSourceLib/Controlled Current Source  Initialize=on  Source_Type=AC  Amplitude=0  Phase=0  Frequency=0  Measurements=None
  Controlled Voltage Source7 : spsControlledVoltageSourceLib/Controlled Voltage Source  Initialize=on  Source_Type=AC  Amplitude=Vdc/2  Phase=0  Frequency=0  Measurements=None
  Current Measurement4 : spsCurrentMeasurementLib/Current Measurement  PhasorSimulation=off  OutputType=Complex  PSBequivalent=0
  Divide1 : Product  Inputs=**
  Divide2 : Product  Inputs=*/
  Filtered Lower arm A instananeous power1 : Scope
  Gain : Gain  Gain=1e6
  Lower arm A instananeous power : Scope
  Series RLC Branch2 : spsSeriesRLCBranchLib/Series RLC Branch  LConnTagsString=__new0  RConnTagsString=__new0  BranchType=C  Resistance=Ra_1  Inductance=La_1  SetiL0=on  InitialCurrent=0  Capacitance=Cap/N  Setx0=on  InitialVoltage=640e3  Measurements=None
  Transfer Fcn : TransferFcn  Denominator=[1 1]
  Voltage Measurement : spsVoltageMeasurementLib/Voltage Measurement  PhasorSimulation=off  OutputType=Complex  PSBequivalent=0
  Conn1 : PMIOPort  Side=Right
  Conn2 : PMIOPort  Port=2  Side=Left
  v_sum_lc : Outport
  wires:
  Gain/1 -> Filtered Lower arm A instananeous power1/1
  Transfer Fcn/1 -> Gain/1
  Current Measurement4/1 -> Divide1/2  "ila"
  Divide1/1 -> Divide2/1, Transfer Fcn/1, Lower arm A instananeous power/1
  Divide2/1 -> Controlled Current Source/1
  Voltage Measurement/1 -> Divide2/2, v_sum_lc/1
  vlc/1 -> Controlled Voltage Source7/1, Divide1/1  "vla"
  connections:
  Conn2/RConn1 -- Current Measurement4/RConn1
  Current Measurement4/LConn1 -- Controlled Voltage Source7/LConn1
  Voltage Measurement/LConn2 -- Series RLC Branch2/RConn1 -- Controlled Current Source/LConn1
  Controlled Current Source/RConn1 -- Series RLC Branch2/LConn1 -- Voltage Measurement/LConn1
  Controlled Voltage Source7/RConn1 -- Conn1/RConn1

== system MMC_SIMULATION (1)/Equivalent arm upper-a ==
  note: Power_ua
  vua : Inport
  Controlled Current Source : spsControlledCurrentSourceLib/Controlled Current Source  Initialize=on  Source_Type=AC  Amplitude=0  Phase=0  Frequency=0  Measurements=None
  Controlled Voltage Source7 : spsControlledVoltageSourceLib/Controlled Voltage Source  Initialize=on  Source_Type=AC  Amplitude=Vdc/2  Phase=0  Frequency=0  Measurements=None
  Current Measurement4 : spsCurrentMeasurementLib/Current Measurement  PhasorSimulation=off  OutputType=Complex  PSBequivalent=0
  Divide1 : Product  Inputs=**
  Divide2 : Product  Inputs=*/
  Filtered Upper arm A instananeous power1 : Scope
  Gain : Gain  Gain=1e6
  Series RLC Branch2 : spsSeriesRLCBranchLib/Series RLC Branch  LConnTagsString=__new0  RConnTagsString=__new0  BranchType=C  Resistance=Ra_1  Inductance=La_1  SetiL0=on  InitialCurrent=0  Capacitance=Cap/N  Setx0=on  InitialVoltage=640e3  Measurements=None
  Transfer Fcn : TransferFcn  Denominator=[1 1]
  Upper arm A instananeous power : Scope
  Voltage Measurement : spsVoltageMeasurementLib/Voltage Measurement  PhasorSimulation=off  OutputType=Complex  PSBequivalent=0
  Conn1 : PMIOPort  Side=Right
  Conn2 : PMIOPort  Port=2  Side=Left
  v_sum_ua : Outport
  wires:
  vua/1 -> Divide1/1, Controlled Voltage Source7/1  "vua"
  Voltage Measurement/1 -> v_sum_ua/1, Divide2/2
  Divide2/1 -> Controlled Current Source/1
  Divide1/1 -> Upper arm A instananeous power/1, Transfer Fcn/1, Divide2/1
  Current Measurement4/1 -> Divide1/2  "iua"
  Transfer Fcn/1 -> Gain/1
  Gain/1 -> Filtered Upper arm A instananeous power1/1
  connections:
  Controlled Voltage Source7/RConn1 -- Conn1/RConn1
  Voltage Measurement/LConn1 -- Series RLC Branch2/LConn1 -- Controlled Current Source/RConn1
  Controlled Current Source/LConn1 -- Series RLC Branch2/RConn1 -- Voltage Measurement/LConn2
  Current Measurement4/LConn1 -- Controlled Voltage Source7/LConn1
  Conn2/RConn1 -- Current Measurement4/RConn1
